simulink model "Single_Phase_VSR_Simulation"  (R2022b)
settings: Solver=FixedStepDiscrete  StartTime=0.0  StopTime=0.6  FixedStep=1e-6  RelTol=1e-3
libraries: spsSeriesRLCBranchLib x10, spsCurrentMeasurementLib x4, spsMosfetLib x4, slpidlib x3, spsRMSLib x3, simulink x3, spsVoltageMeasurementLib x3, spsFourierLib x2, spsMeanLib x2, spsIdealSwitchLib x1, spspowerguiLib x1, spsControlledVoltageSourceLib x1
(part 1 of 2)
settings Model: Creator=XIAO  LastModifiedBy=XIAO
settings SolverCC: AutoInsertRateTranBlk=on
settings DataIOCC: ReturnWorkspaceOutputs=off

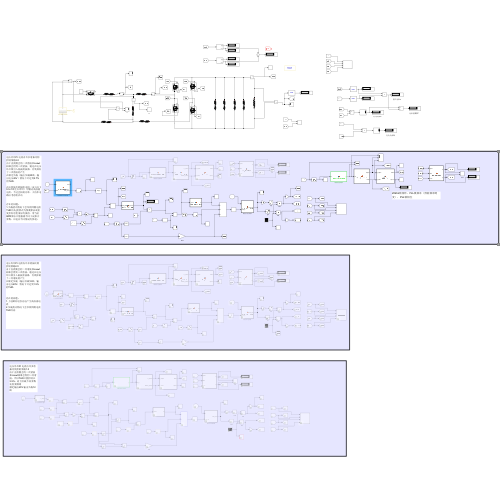
[thumbnail: Simulink's stored preview of the top-level diagram]
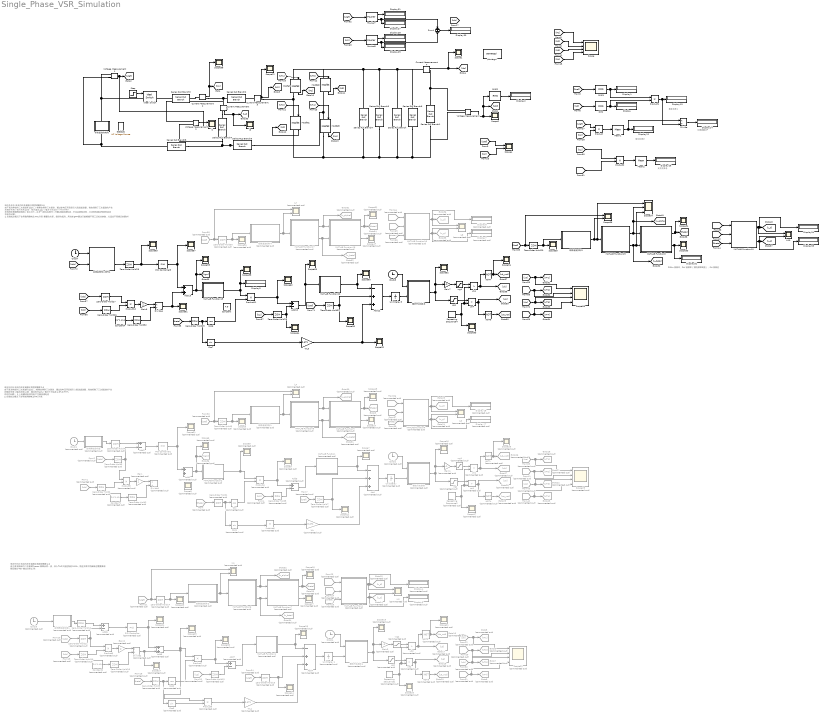
== system Single_Phase_VSR_Simulation ==
  note: 功率因数PF
  note: 有功功率P
  note: 电压外环PI 电流内环多谐振比例控制策略2.0
      | 由于直流侧会的二次谐波和coswt相乘会得到三次谐波，通过在电压环后级引入陷波滤波器，有效抑制了三次谐波的产生
      | 在额定负载（输出负载12欧，输出电压40V）情况下可达到1.5%的THD。
      |
      | 存在的问题：
      | 1.上电瞬间电容充电产生高浪涌电流
      | 2.负载扰动情况下会导致网侧电流THD升高
  note: 无功功率Q
  note: 视在功率s
  note: 电压外环PI 电流内环多谐振比例控制策略1.0
      | 由于直流侧会的二次谐波和coswt相乘会得到三次谐波，所以THD只能控制在3.5%，而且负载不同参数还需要微调
      | 额定输出40V 输出负载12欧
  note: 电压外环PI 电流内环多谐振比例控制策略3.0
      | 由于直流侧会的二次谐波和coswt相乘会得到三次谐波，通过在电压环后级引入陷波滤波器，有效抑制了三次谐波的产生
      | 在额定负载（输出负载20欧，输出电压40V）情况下可达到2.7%的THD。
      |
      | 在电网处串联限流电阻（该工况下0.5~1欧左右即可）可解决高浪涌电流，不过会损耗功率，大功率电路应考虑软启动
      |
      | 存在的问题：
      | 1.负载扰动情况下会导致网侧电流THD升高(需要改为预测算法或重复控制才能很好的抵消，用当前QPR算法只能根据不同工况拟合参数，以适应不同情况的要求)
  note: 20khz锁相环，FLL锁频率（预防频率畸变），PLL锁相位
  -ug1 : Saturate  Commented=on  UpperLimit=1  LowerLimit=-1
  -ug2 : Saturate  Commented=on  UpperLimit=1  LowerLimit=-1
  -ug4 : Saturate  UpperLimit=1  LowerLimit=-1
  Add : Sum  Commented=on  Inputs=-++
  Add1 : Sum  Commented=on
  Add10 : Sum  Inputs=+-
  Add12 : Sum  Inputs=-++
  Add13 : Sum
  Add{2..3,6..7} (4 alike) : Sum  Commented=on  Inputs=+-
  Add4 : Sum  Commented=on  Inputs=-++
  Add5 : Sum  Commented=on
  Clock{1..4} (4 alike) : Clock  Commented=on
  Clock7 : Clock
  Clock8 : Clock
  Constant : Constant  Value=4.9
  Constant1 : Constant  Commented=on  Value=24*1.414
  Constant2 : Constant  Commented=on  Value=24*1.414
  Constant4 : Constant  Value=24*1.414
  Cos : Trigonometry  Commented=on  Operator=cos
  Cos1 : Trigonometry  Commented=on
  Cos2 : Trigonometry  Commented=on  Operator=cos
  Cos3 : Trigonometry  Commented=on
  Cos6 : Trigonometry  Operator=cos
  Cos7 : Trigonometry
  Current Measurement{1..4} (4 alike) : spsCurrentMeasurementLib/Current Measurement  PhasorSimulation=off  OutputType=Complex  PSBequivalent=0
  Display{,1..2,5,12..14,26..34} (16 alike) : Display
  Display{3..4,7..8,17..18} (6 alike) : Display  Commented=on
  Divide : Product  Inputs=*/
  Divide1 : Product  Commented=on  Inputs=*/
  Divide2 : Product  Commented=on  Inputs=*/
  Divide4 : Product  Inputs=*/
  Fourier7 : spsFourierLib/Fourier  Freq=50  n=1  InInit=[0, 0]  Ts=1e-6
  Fourier8 : spsFourierLib/Fourier  Freq=50  n=1  InInit=[0, 0]  Ts=1e-6
  From{,18,25,39,66} (5 alike) : From  Commented=on  GotoTag=theta
  From1 : From  Commented=on  GotoTag=Idc
  From19 : From  Commented=on  GotoTag=Idc
  From2 : From  Commented=on  GotoTag=Udc
  From20 : From  Commented=on  GotoTag=Udc
  From{7,21,30,34,58} (5 alike) : From  Commented=on  GotoTag=Uref
  From22 : From  Commented=on  GotoTag=ua
  From23 : From  Commented=on  GotoTag=u_alpha
  From24 : From  Commented=on  GotoTag=u_beta
  From26 : From  Commented=on  GotoTag=IL2
  From29 : From  Commented=on  GotoTag=ua_not
  From31 : From  Commented=on  GotoTag=ub_not
  From32 : From  Commented=on  GotoTag=ub
  From33 : From  Commented=on  GotoTag=ua
  From36 : From  Commented=on  GotoTag=u_alpha
  From37 : From  Commented=on  GotoTag=u_beta
  From4 : From  Commented=on  GotoTag=IL2
  From41 : From  Commented=on  GotoTag=ua_not
  From42 : From  Commented=on  GotoTag=ub_not
  From43 : From  Commented=on  GotoTag=ub
  From64 : From  Commented=on  GotoTag=u_alpha
  From65 : From  Commented=on  GotoTag=u_beta
  Gain : Gain  Commented=on  Gain=2
  Gain1 : Gain  Commented=on  Gain=-1
  Gain2 : Gain  Commented=on  Gain=2
  Gain3 : Gain  Commented=on  Gain=-1
  Gain6 : Gain  Gain=2
  Gain7 : Gain  Gain=-1
  Goto14 : Goto  Commented=on  GotoTag=u_q
  Goto15 : Goto  Commented=on  GotoTag=u_d
  Goto16 : Goto  Commented=on  GotoTag=ub_not
  Goto17 : Goto  Commented=on  GotoTag=ub
  Goto18 : Goto  Commented=on  GotoTag=VT1
  Goto19 : Goto  Commented=on  GotoTag=ua
  Goto20 : Goto  Commented=on  GotoTag=ua_not
  Goto21 : Goto  Commented=on  GotoTag=VT2
  Goto22 : Goto  Commented=on  GotoTag=VT3
  Goto23 : Goto  Commented=on  GotoTag=VT4
  Goto24 : Goto  Commented=on  GotoTag=u_q
  Goto25 : Goto  Commented=on  GotoTag=u_d
  Goto26 : Goto  Commented=on  GotoTag=ub_not
  Goto27 : Goto  Commented=on  GotoTag=ub
  Goto28 : Goto  Commented=on  GotoTag=ua
  Goto29 : Goto  Commented=on  GotoTag=ua_not
  Goto30 : Goto  Commented=on  GotoTag=u_alpha
  Goto31 : Goto  Commented=on  GotoTag=u_beta
  Goto32 : Goto  Commented=on  GotoTag=u_alpha
  Goto34 : Goto  Commented=on  GotoTag=u_beta
  Goto35 : Goto  Commented=on  GotoTag=theta
  Goto36 : Goto  Commented=on  GotoTag=Igm
  Goto5 : Goto  Commented=on  GotoTag=VT1
  Goto55 : Goto  Commented=on  GotoTag=u_q
  Goto56 : Goto  Commented=on  GotoTag=u_d
  Goto6 : Goto  Commented=on  GotoTag=VT2
  Goto61 : Goto  Commented=on  GotoTag=u_alpha
  Goto62 : Goto  Commented=on  GotoTag=u_beta
  Goto64 : Goto  Commented=on  GotoTag=theta
  Goto7 : Goto  Commented=on  GotoTag=VT3
  Goto8 : Goto  Commented=on  GotoTag=VT4
  Goto9 : Goto  Commented=on  GotoTag=theta
  Ideal Switch : spsIdealSwitchLib/Ideal Switch  Ron=0.001  Lon=0  IC=0  Rs=1e5  Cs=inf  Measurements=on
  MATLAB Function : MATLAB Function  Commented=on  TreatAsAtomicUnit=on
  MATLAB Function1 : MATLAB Function  Commented=on  TreatAsAtomicUnit=on
  MATLAB Function10 : MATLAB Function  TreatAsAtomicUnit=on
  MATLAB Function15 : MATLAB Function  TreatAsAtomicUnit=on
  MATLAB Function16 : MATLAB Function  Commented=on  TreatAsAtomicUnit=on
  MATLAB Function17 : MATLAB Function  Commented=on  TreatAsAtomicUnit=on
  MATLAB Function18 : MATLAB Function  Commented=on  TreatAsAtomicUnit=on
  MATLAB Function19 : MATLAB Function  TreatAsAtomicUnit=on
  MATLAB Function2 : MATLAB Function  Commented=on  TreatAsAtomicUnit=on
  MATLAB Function20 : MATLAB Function  TreatAsAtomicUnit=on
  MATLAB Function3 : MATLAB Function  TreatAsAtomicUnit=on
  MATLAB Function4 : MATLAB Function  Commented=on  TreatAsAtomicUnit=on
  MATLAB Function5 : MATLAB Function  Commented=on  TreatAsAtomicUnit=on
  MATLAB Function6 : MATLAB Function  Commented=on  TreatAsAtomicUnit=on
  MATLAB Function7 : MATLAB Function  Commented=on  TreatAsAtomicUnit=on
  MATLAB Function8 : MATLAB Function  Commented=on  TreatAsAtomicUnit=on
  MATLAB Function9 : MATLAB Function  Commented=on  TreatAsAtomicUnit=on
  Mean1 : spsMeanLib/Mean  Freq=50  Vinit=0  Ts=5e-5
  Mean2 : spsMeanLib/Mean  Freq=50  Vinit=0  Ts=5e-5
  Mosfet{,1..3} (4 alike) : spsMosfetLib/Mosfet  Ron=0.1  Lon=0  Rd=0.01  Vfd=0  IC=0  Rs=1e5  Cs=inf  Measurements=on
  NOT{1..4} (4 alike) : Logic  Commented=on  Operator=NOT  IconShape=distinctive  AllPortsSameDT=off  OutDataTypeStr=boolean
  NOT7 : Logic  Operator=NOT  IconShape=distinctive  AllPortsSameDT=off  OutDataTypeStr=boolean
  NOT8 : Logic  Operator=NOT  IconShape=distinctive  AllPortsSameDT=off  OutDataTypeStr=boolean
  PID Controller : slpidlib/PID Controller  Commented=on  Controller=PI  Form=Parallel  TimeDomain=Discrete-time  UseExternalTs=off  SampleTime=-1  IntegratorMethod=Forward Euler  FilterMethod=Forward Euler  ControllerParametersSource=internal  P=0.5  I=10  UseKiTs=off  D=0  N=100  UseFilter=on  TunerSelectOption=Transfer Function Based (PID Tuner App)  InitialConditionSource=internal  InitialConditionForIntegrator=0  InitialConditionForFilter=0  DifferentiatorICPrevScaledInput=0  ExternalReset=none  TrackingMode=off  Kt=1  LimitOutput=off  SatLimitsSource=internal  UpperSaturationLimit=inf  LowerSaturationLimit=-inf  LinearizeAsGain=on  AntiWindupMode=none  Kb=1  LimitIntegrator=off  UpperIntegratorSaturationLimit=inf  LowerIntegratorSaturationLimit=-inf  POutMin=[]  POutMax=[]  IOutMin=[]  IOutMax=[]  DOutMin=[]  DOutMax=[]  NOutMin=[]  NOutMax=[]  SumOutMin=[]  SumOutMax=[]  SaturationOutMin=[]  SaturationOutMax=[]  PParamMin=[]  PParamMax=[]  IParamMin=[]  IParamMax=[]  DParamMin=[]  DParamMax=[]  NParamMin=[]  NParamMax=[]  KbParamMin=[]  KbParamMax=[]  KtParamMin=[]  KtParamMax=[]  KbOutMin=[]  KbOutMax=[]  KtOutMin=[]  KtOutMax=[]  IntegratorOutMin=[]  IntegratorOutMax=[]  FilterOutMin=[]  FilterOutMax=[]  SumI1OutMin=[]  SumI1OutMax=[]  SumI2OutMin=[]  SumI2OutMax=[]  SumI3OutMin=[]  SumI3OutMax=[]  SumI4OutMin=[]  SumI4OutMax=[]  SumDOutMin=[]  SumDOutMax=[]  DifferentiatorOutMin=[]  DifferentiatorOutMax=[]  FilterDiffOutCoefMin=[]  FilterDiffOutCoefMax=[]  ReciprocalOutMin=[]  ReciprocalOutMax=[]  SumDenOutMin=[]  SumDenOutMax=[]  SumNumOutMin=[]  SumNumOutMax=[]  DivideOutMin=[]  DivideOutMax=[]  UdiffTsProdOutMin=[]  UdiffTsProdOutMax=[]  NTsProdOutMin=[]  NTsProdOutMax=[]  UintegralTsProdOutMin=[]  UintegralTsProdOutMax=[]  UngainTsProdOutMin=[]  UngainTsProdOutMax=[]  ClampingZeroOutDataTypeStr=Inherit: Inherit via back propagation  ClampingZeroOutMin=[]  ClampingZeroOutMax=[]  FilterDenConstantOutDataTypeStr=Inherit: Inherit via back propagation  FilterDenConstantOutMin=[]  FilterDenConstantOutMax=[]  PCopyOutDataTypeStr=Inherit: Inherit via back propagation  PCopyOutMin=[]  PCopyOutMax=[]  NCopyOutDataTypeStr=Inherit: Inherit via back propagation  NCopyOutMin=[]  NCopyOutMax=[]  IntegratorContinuousStateAttributes=''  IntegratorStateMustResolveToSignalObject=off  IntegratorRTWStateStorageClass=Auto  FilterContinuousStateAttributes=''  FilterStateMustResolveToSignalObject=off  FilterRTWStateStorageClass=Auto  ParallelPVariant=InternalParameters  IdealPVariant=Disabled  IVariant=InternalParameters  DVariant=Disabled  IntegratorVariant=Discrete  SatVariant=Disabled  AWVariant=Passthrough  PCopyVariant=Disabled  TRVariant=Disabled  FdbkBlocksVariant=Forward  IdealPFdbkVariant=Disabled  SatFdbkVariant=Disabled  DerivativeFilterVariant=Disabled  NVariant=Disabled  NCopyVariant=Disabled_SignalSpec  FilterICVariant=Disabled  IntegratorICVariant=InternalICs  ExternalResetVariant=Disabled  TRSumVariant=Passthrough  SumFdbkVariant=Disabled  SumVariant=Sum_PI  TsampFilterVariant=InternalTs  TsampNgainVariant=Passthrough  TsampIntegralVariant=Passthrough  ExternalSaturationOutDataTypeStr=Inherit: Same as second input
  PID Controller1 : slpidlib/PID Controller  Commented=on  Controller=PI  Form=Parallel  TimeDomain=Discrete-time  UseExternalTs=off  SampleTime=-1  IntegratorMethod=Forward Euler  FilterMethod=Forward Euler  ControllerParametersSource=internal  P=0.5  I=10  UseKiTs=off  D=0  N=100  UseFilter=on  TunerSelectOption=Transfer Function Based (PID Tuner App)  InitialConditionSource=internal  InitialConditionForIntegrator=0  InitialConditionForFilter=0  DifferentiatorICPrevScaledInput=0  ExternalReset=none  TrackingMode=off  Kt=1  LimitOutput=off  SatLimitsSource=internal  UpperSaturationLimit=inf  LowerSaturationLimit=-inf  LinearizeAsGain=on  AntiWindupMode=none  Kb=1  LimitIntegrator=off  UpperIntegratorSaturationLimit=inf  LowerIntegratorSaturationLimit=-inf  POutMin=[]  POutMax=[]  IOutMin=[]  IOutMax=[]  DOutMin=[]  DOutMax=[]  NOutMin=[]  NOutMax=[]  SumOutMin=[]  SumOutMax=[]  SaturationOutMin=[]  SaturationOutMax=[]  PParamMin=[]  PParamMax=[]  IParamMin=[]  IParamMax=[]  DParamMin=[]  DParamMax=[]  NParamMin=[]  NParamMax=[]  KbParamMin=[]  KbParamMax=[]  KtParamMin=[]  KtParamMax=[]  KbOutMin=[]  KbOutMax=[]  KtOutMin=[]  KtOutMax=[]  IntegratorOutMin=[]  IntegratorOutMax=[]  FilterOutMin=[]  FilterOutMax=[]  SumI1OutMin=[]  SumI1OutMax=[]  SumI2OutMin=[]  SumI2OutMax=[]  SumI3OutMin=[]  SumI3OutMax=[]  SumI4OutMin=[]  SumI4OutMax=[]  SumDOutMin=[]  SumDOutMax=[]  DifferentiatorOutMin=[]  DifferentiatorOutMax=[]  FilterDiffOutCoefMin=[]  FilterDiffOutCoefMax=[]  ReciprocalOutMin=[]  ReciprocalOutMax=[]  SumDenOutMin=[]  SumDenOutMax=[]  SumNumOutMin=[]  SumNumOutMax=[]  DivideOutMin=[]  DivideOutMax=[]  UdiffTsProdOutMin=[]  UdiffTsProdOutMax=[]  NTsProdOutMin=[]  NTsProdOutMax=[]  UintegralTsProdOutMin=[]  UintegralTsProdOutMax=[]  UngainTsProdOutMin=[]  UngainTsProdOutMax=[]  ClampingZeroOutDataTypeStr=Inherit: Inherit via back propagation  ClampingZeroOutMin=[]  ClampingZeroOutMax=[]  FilterDenConstantOutDataTypeStr=Inherit: Inherit via back propagation  FilterDenConstantOutMin=[]  FilterDenConstantOutMax=[]  PCopyOutDataTypeStr=Inherit: Inherit via back propagation  PCopyOutMin=[]  PCopyOutMax=[]  NCopyOutDataTypeStr=Inherit: Inherit via back propagation  NCopyOutMin=[]  NCopyOutMax=[]  IntegratorContinuousStateAttributes=''  IntegratorStateMustResolveToSignalObject=off  IntegratorRTWStateStorageClass=Auto  FilterContinuousStateAttributes=''  FilterStateMustResolveToSignalObject=off  FilterRTWStateStorageClass=Auto  ParallelPVariant=InternalParameters  IdealPVariant=Disabled  IVariant=InternalParameters  DVariant=Disabled  IntegratorVariant=Discrete  SatVariant=Disabled  AWVariant=Passthrough  PCopyVariant=Disabled  TRVariant=Disabled  FdbkBlocksVariant=Forward  IdealPFdbkVariant=Disabled  SatFdbkVariant=Disabled  DerivativeFilterVariant=Disabled  NVariant=Disabled  NCopyVariant=Disabled_SignalSpec  FilterICVariant=Disabled  IntegratorICVariant=InternalICs  ExternalResetVariant=Disabled  TRSumVariant=Passthrough  SumFdbkVariant=Disabled  SumVariant=Sum_PI  TsampFilterVariant=InternalTs  TsampNgainVariant=Passthrough  TsampIntegralVariant=Passthrough  ExternalSaturationOutDataTypeStr=Inherit: Same as second input
  PID Controller3 : slpidlib/PID Controller  Controller=PI  Form=Parallel  TimeDomain=Discrete-time  UseExternalTs=off  SampleTime=-1  IntegratorMethod=Forward Euler  FilterMethod=Forward Euler  ControllerParametersSource=internal  P=0.5  I=10  UseKiTs=off  D=0  N=100  UseFilter=on  TunerSelectOption=Transfer Function Based (PID Tuner App)  InitialConditionSource=internal  InitialConditionForIntegrator=0  InitialConditionForFilter=0  DifferentiatorICPrevScaledInput=0  ExternalReset=none  TrackingMode=off  Kt=1  LimitOutput=off  SatLimitsSource=internal  UpperSaturationLimit=inf  LowerSaturationLimit=-inf  LinearizeAsGain=on  AntiWindupMode=none  Kb=1  LimitIntegrator=off  UpperIntegratorSaturationLimit=inf  LowerIntegratorSaturationLimit=-inf  POutMin=[]  POutMax=[]  IOutMin=[]  IOutMax=[]  DOutMin=[]  DOutMax=[]  NOutMin=[]  NOutMax=[]  SumOutMin=[]  SumOutMax=[]  SaturationOutMin=[]  SaturationOutMax=[]  PParamMin=[]  PParamMax=[]  IParamMin=[]  IParamMax=[]  DParamMin=[]  DParamMax=[]  NParamMin=[]  NParamMax=[]  KbParamMin=[]  KbParamMax=[]  KtParamMin=[]  KtParamMax=[]  KbOutMin=[]  KbOutMax=[]  KtOutMin=[]  KtOutMax=[]  IntegratorOutMin=[]  IntegratorOutMax=[]  FilterOutMin=[]  FilterOutMax=[]  SumI1OutMin=[]  SumI1OutMax=[]  SumI2OutMin=[]  SumI2OutMax=[]  SumI3OutMin=[]  SumI3OutMax=[]  SumI4OutMin=[]  SumI4OutMax=[]  SumDOutMin=[]  SumDOutMax=[]  DifferentiatorOutMin=[]  DifferentiatorOutMax=[]  FilterDiffOutCoefMin=[]  FilterDiffOutCoefMax=[]  ReciprocalOutMin=[]  ReciprocalOutMax=[]  SumDenOutMin=[]  SumDenOutMax=[]  SumNumOutMin=[]  SumNumOutMax=[]  DivideOutMin=[]  DivideOutMax=[]  UdiffTsProdOutMin=[]  UdiffTsProdOutMax=[]  NTsProdOutMin=[]  NTsProdOutMax=[]  UintegralTsProdOutMin=[]  UintegralTsProdOutMax=[]  UngainTsProdOutMin=[]  UngainTsProdOutMax=[]  ClampingZeroOutDataTypeStr=Inherit: Inherit via back propagation  ClampingZeroOutMin=[]  ClampingZeroOutMax=[]  FilterDenConstantOutDataTypeStr=Inherit: Inherit via back propagation  FilterDenConstantOutMin=[]  FilterDenConstantOutMax=[]  PCopyOutDataTypeStr=Inherit: Inherit via back propagation  PCopyOutMin=[]  PCopyOutMax=[]  NCopyOutDataTypeStr=Inherit: Inherit via back propagation  NCopyOutMin=[]  NCopyOutMax=[]  IntegratorContinuousStateAttributes=''  IntegratorStateMustResolveToSignalObject=off  IntegratorRTWStateStorageClass=Auto  FilterContinuousStateAttributes=''  FilterStateMustResolveToSignalObject=off  FilterRTWStateStorageClass=Auto  ParallelPVariant=InternalParameters  IdealPVariant=Disabled  IVariant=InternalParameters  DVariant=Disabled  IntegratorVariant=Discrete  SatVariant=Disabled  AWVariant=Passthrough  PCopyVariant=Disabled  TRVariant=Disabled  FdbkBlocksVariant=Forward  IdealPFdbkVariant=Disabled  SatFdbkVariant=Disabled  DerivativeFilterVariant=Disabled  NVariant=Disabled  NCopyVariant=Disabled_SignalSpec  FilterICVariant=Disabled  IntegratorICVariant=InternalICs  ExternalResetVariant=Disabled  TRSumVariant=Passthrough  SumFdbkVariant=Disabled  SumVariant=Sum_PI  TsampFilterVariant=InternalTs  TsampNgainVariant=Passthrough  TsampIntegralVariant=Passthrough  ExternalSaturationOutDataTypeStr=Inherit: Same as second input
  Product{,1..2,11..12} (5 alike) : Product
  Product{3..8} (6 alike) : Product  Commented=on
  RMS : spsRMSLib/RMS  TrueRMS=on  Freq=50  RMSInit=24  Ts=1e-6
  RMS1 : spsRMSLib/RMS  TrueRMS=on  Freq=50  RMSInit=24  Ts=1e-6
  RMS2 : spsRMSLib/RMS  TrueRMS=on  Freq=50  RMSInit=24  Ts=1e-6
  Repeating Sequence1 : simulink/Sources/Repeating Sequence  Commented=on  rep_seq_t=[0, 5e-5, 1e-4]  rep_seq_y=[-1, 1, -1]
  Repeating Sequence2 : simulink/Sources/Repeating Sequence  Commented=on  rep_seq_t=[0, 5e-5, 1e-4]  rep_seq_y=[-1, 1, -1]
  Repeating Sequence4 : simulink/Sources/Repeating Sequence  rep_seq_t=[0, 5e-5, 1e-4]  rep_seq_y=[-1, 1, -1]
  Scope : Scope  NumInputPorts=4
  Scope{1..2,12,32..35,38,50,52,54,57..65} (20 alike) : Scope
  Scope{3,5..11,13..16,18..19,21,23..28,30..31,49,51,56} (26 alike) : Scope  Commented=on
  Scope17 : Scope  Commented=on  NumInputPorts=2
  Scope20 : Scope  Commented=on  NumInputPorts=2
  Scope22 : Scope  Commented=on  NumInputPorts=4
  Scope29 : Scope  Commented=on  NumInputPorts=4
  Scope36 : Scope  NumInputPorts=2
  Scope37 : Scope  NumInputPorts=3
  Scope4 : Scope  NumInputPorts=2
  Scope53 : Scope  NumInputPorts=2
  Scope55 : Scope  NumInputPorts=4
  Series RLC Branch{,5..7} (4 alike) : spsSeriesRLCBranchLib/Series RLC Branch  LConnTagsString=__new0  RConnTagsString=__new0  BranchType=RC  Resistance=0.01  Inductance=0  SetiL0=off  InitialCurrent=0  Capacitance=470e-6  Setx0=off  InitialVoltage=0  Measurements=None
  Series RLC Branch1 : spsSeriesRLCBranchLib/Series RLC Branch  LConnTagsString=__new0  RConnTagsString=__new0  BranchType=R  Resistance=20  Inductance=0  SetiL0=off  InitialCurrent=0  Capacitance=470e-6  Setx0=off  InitialVoltage=0  Measurements=None
  Series RLC Branch2 : spsSeriesRLCBranchLib/Series RLC Branch  LConnTagsString=__new0  RConnTagsString=__new0  BranchType=RL  Resistance=0.1  Inductance=0.0015  SetiL0=off  InitialCurrent=0  Capacitance=220e-6  Setx0=off  InitialVoltage=0  Measurements=None
  Series RLC Branch3 : spsSeriesRLCBranchLib/Series RLC Branch  LConnTagsString=__new0  RConnTagsString=__new0  BranchType=RL  Resistance=0.1  Inductance=0.00012  SetiL0=off  InitialCurrent=0  Capacitance=220e-6  Setx0=off  InitialVoltage=0  Measurements=None
  Series RLC Branch4 : spsSeriesRLCBranchLib/Series RLC Branch  LConnTagsString=__new0  RConnTagsString=__new0  BranchType=RC  Resistance=0.1  Inductance=0  SetiL0=off  InitialCurrent=0  Capacitance=10e-6  Setx0=off  InitialVoltage=0  Measurements=None
  Series RLC Branch8 : spsSeriesRLCBranchLib/Series RLC Branch  LConnTagsString=__new0  RConnTagsString=__new0  BranchType=RL  Resistance=0.1  Inductance=0.00012  SetiL0=off  InitialCurrent=0  Capacitance=220e-6  Setx0=off  InitialVoltage=0  Measurements=None
  Series RLC Branch9 : spsSeriesRLCBranchLib/Series RLC Branch  LConnTagsString=__new0  RConnTagsString=__new0  BranchType=RL  Resistance=0.1  Inductance=0.0015  SetiL0=off  InitialCurrent=0  Capacitance=220e-6  Setx0=off  InitialVoltage=0  Measurements=None
  Step : Step  Time=0.15  SampleTime=1e-6
  Sum4 : Sum  Inputs=+-
  Unit Delay : UnitDelay  Commented=on  SampleTime=5e-5  HasFrameUpgradeWarning=on
  Unit Delay1 : UnitDelay  Commented=on  SampleTime=5e-5  HasFrameUpgradeWarning=on
  Unit Delay3 : UnitDelay  SampleTime=5e-5  HasFrameUpgradeWarning=on
  Voltage Measurement : spsVoltageMeasurementLib/Voltage Measurement  PhasorSimulation=off  OutputType=Complex  PSBequivalent=0
  Voltage Measurement1 : spsVoltageMeasurementLib/Voltage Measurement  PhasorSimulation=off  OutputType=Complex  PSBequivalent=0
  Voltage Measurement2 : spsVoltageMeasurementLib/Voltage Measurement  PhasorSimulation=off  OutputType=Complex  PSBequivalent=0
  WL : Gain  Commented=on  Gain=0.471
  WL1 : Gain  Commented=on  Gain=0.471
  WL3 : Gain  Gain=0.471
  Zero-Order Hold{1..5,7..13,15..16} (14 alike) : ZeroOrderHold  Commented=on  SampleTime=5e-5
  Zero-Order Hold14 : ZeroOrderHold  Commented=on  SampleTime=1e-5
  Zero-Order Hold{20,25..29,31..32} (8 alike) : ZeroOrderHold  SampleTime=5e-5
  Zero-Order Hold30 : ZeroOrderHold  Commented=on  SampleTime=1e-5
  Zero-Order Hold6 : ZeroOrderHold  Commented=on  SampleTime=1e-5
  i1 : Scope  NumInputPorts=2
  i3 : Scope
  iL{1..2,4..5,7..8} (6 alike) : Scope  Commented=on  NumInputPorts=2
  iL10 : Scope  NumInputPorts=2
  powergui : spspowerguiLib/powergui  Priority=1  SimulationMode=Discrete  SampleTime=1e-6  frequency=60  Iterations=50  frequencyindice=0  Pbase=100e6  ErrMax=1e-4  UnitsV=kV  UnitsW=MW  buscounter=0  FunctionMessages=off  echomessages=off  EnableUseOfTLC=off  CurrentSourceSwitches=off  DisableSnubberDevices=off  DisableRonSwitches=off  DisableVfSwitches=off  DisplayEquations=off  AutomaticDiscreteSolvers=off  SolverType=Tustin/Backward Euler (TBE)  Interpol=off  ExternalGateDelay=off  methode=off  Ts=100  x0status=blocks  SPID=on  SwTol=0  HookPort=off  NonlinearTolerance=1e-4  nMaxIteration=100  ContinueOnMaxIteration=off  RestoreLinks=warning  ResistiveCurrentMeasurement=off  Frange=[0:2:500]  Ylog=off  Xlog=on  ShowGrid=off  save=off  variable=ZData  structure=0  ZoomFFT=off  StartTime=0.0  cycles=1  DisplayStyle=1  fundamental=60  FreqAxis=off  MaxFrequency=1000  frequencyindicesteady=1  RmsSteady=1  display=off
  ua1 : RelationalOperator  Commented=on  Operator=>  OutDataTypeStr=boolean  RndMeth=Simplest  InputSameDT=off
  ua2 : RelationalOperator  Commented=on  Operator=>  OutDataTypeStr=boolean  RndMeth=Simplest  InputSameDT=off
  ua4 : RelationalOperator  Operator=>  OutDataTypeStr=boolean  RndMeth=Simplest  InputSameDT=off
  ub1 : RelationalOperator  Commented=on  Operator=>  OutDataTypeStr=boolean  RndMeth=Simplest  InputSameDT=off
  ub2 : RelationalOperator  Commented=on  Operator=>  OutDataTypeStr=boolean  RndMeth=Simplest  InputSameDT=off
  ub4 : RelationalOperator  Operator=>  OutDataTypeStr=boolean  RndMeth=Simplest  InputSameDT=off
  ug1 : Saturate  Commented=on  UpperLimit=1  LowerLimit=-1
  ug2 : Saturate  Commented=on  UpperLimit=1  LowerLimit=-1
  ug4 : Saturate  UpperLimit=1  LowerLimit=-1
  合闸再给目标值 : MATLAB Function  Commented=on  TreatAsAtomicUnit=on
  合闸再给目标值1 : MATLAB Function  Commented=on  TreatAsAtomicUnit=on
  合闸后再传入信号1 : MATLAB Function  TreatAsAtomicUnit=on
  带有谐波的电网 : Subsystem
  模仿开关控制 : MATLAB Function  Commented=on  TreatAsAtomicUnit=on
  模仿开关控制1 : MATLAB Function  Commented=on  TreatAsAtomicUnit=on
  模仿开关控制3 : MATLAB Function  TreatAsAtomicUnit=on
  理想电网 : spsACVoltageSourceLib/AC Voltage Source  Amplitude=24*1.414  Phase=0  Frequency=50  SampleTime=0  Measurements=None  BusType=swing  Pref=10e3  Qref=0  Qmin=-inf  Qmax=+inf
  级联谐波抑制1 : MATLAB Function  Commented=on  TreatAsAtomicUnit=on
  级联谐波抑制2 : MATLAB Function  Commented=on  TreatAsAtomicUnit=on
  级联谐波抑制3 : MATLAB Function  TreatAsAtomicUnit=on
  级联谐波抑制4 : MATLAB Function  Commented=on  TreatAsAtomicUnit=on
  wires:
  Repeating Sequence2/1 -> ub1/2, ua1/2, Scope17/1
  [Uref] -> Fourier7/1
  Mean2/1 -> Display26/1
  Sum4/1 -> Display30/1
  [VT1] -> Mosfet/1
  [IL2] -> Fourier8/1
  Fourier8/2 -> Sum4/2, Display29/1
  Fourier8/1 -> Display28/1
  ua1/1 -> Goto28/1, NOT4/1
  [u_beta] -> Product2/2
  Fourier7/2 -> Display27/1, Sum4/1
  [IL2] -> RMS/1
  [IL2] -> Product2/1
  From33/1 -> Scope29/1, Goto18/1
  [M1] -> Scope/1
  Product2/1 -> Mean2/1
  From36/1 -> MATLAB Function5/1(alpha)
  [Uref] -> Product/1
  Mosfet3/1 -> [M4]
  From43/1 -> Scope29/3, Goto22/1
  [M4] -> Scope/4
  RMS1/1 -> Product1/1, Display1/1
  Gain1/1 -> -ug1/1
  Product1/1 -> Divide/2, Display13/1
  MATLAB Function9/2(qerror) -> Scope10/1
  Divide/1 -> Display14/1
  Mosfet2/1 -> [M3]
  [VT4] -> Mosfet3/1
  ug1/1 -> ua1/1
  Mean1/1 -> Divide/1, Display12/1
  Mosfet/1 -> [M1]
  Mosfet1/1 -> [M2]
  [M3] -> Scope/3
  [VT2] -> Mosfet1/1
  RMS/1 -> Product1/2, Display/1
  [Uref] -> RMS1/1
  NOT1/1 -> Scope28/1, Goto26/1
  [VT3] -> Mosfet2/1
  Fourier7/1 -> Display31/1
  Voltage Measurement1/1 -> i1/2, [Uref]
  级联谐波抑制1/1(y) -> iL4/2, MATLAB Function8/1(U_in)
  -ug1/1 -> ub1/1
  From41/1 -> Scope29/2, Goto21/1
  From42/1 -> Scope29/4, Goto23/1
  ub1/1 -> Goto27/1, NOT1/1
  MATLAB Function5/2(q) -> Display17/1, Goto24/1, iL5/2
  MATLAB Function8/2(deltaU_prime) -> Goto31/1, MATLAB Function9/2(u_beta)
  Product/1 -> Mean1/1
  NOT4/1 -> Goto29/1
  [M2] -> Scope/2
  Current Measurement1/1 -> i3/1, [I_c]
  [IL2] -> Product/2
  From30/1 -> iL4/1, Zero-Order Hold6/1
  MATLAB Function8/1(U_prime) -> MATLAB Function9/1(u_alpha), Goto30/1
  From37/1 -> MATLAB Function5/2(beta)
  From39/1 -> MATLAB Function5/3(theta)
  MATLAB Function5/1(d) -> iL5/1, Display18/1, Goto25/1
  Zero-Order Hold6/1 -> 级联谐波抑制1/1(u), Scope3/1
  MATLAB Function9/1(theta) -> Scope15/1, Goto9/1
  Voltage Measurement/1 -> [Udc], RMS2/1, Scope2/1
  RMS2/1 -> Display2/1
  Current Measurement2/1 -> Scope38/1, [IL1]
  Current Measurement3/1 -> [IL2], Scope12/1
  From/1 -> Zero-Order Hold1/1
  Zero-Order Hold1/1 -> Cos1/1, Cos/1
  Current Measurement4/1 -> Scope1/1, [Idc]
  From1/1 -> Zero-Order Hold2/1
  From2/1 -> Zero-Order Hold3/1
  Zero-Order Hold4/1 -> Add2/1
  Zero-Order Hold3/1 -> Product3/1, Add2/2
  Zero-Order Hold2/1 -> Product3/2
  Product3/1 -> Gain/1
  Gain/1 -> Divide1/1
  Cos/1 -> Product4/2
  Product4/1 -> Scope9/1, Add3/1
  From4/1 -> Zero-Order Hold5/1
  Zero-Order Hold5/1 -> Add3/2
  Add3/1 -> MATLAB Function/1(i_error)
  From7/1 -> Zero-Order Hold7/1
  Zero-Order Hold7/1 -> Add/2, Scope11/1
  Cos1/1 -> Product5/2
  Product5/1 -> WL/1
  Constant1/1 -> Zero-Order Hold8/1
  Zero-Order Hold8/1 -> Divide1/2
  [IL2] -> Scope4/2
  [Uref] -> Scope4/1
  MATLAB Function/1(m) -> Add/1, Scope7/1
  Step/1 -> Ideal Switch/1
  Clock1/1 -> 合闸再给目标值/1(t)
  合闸再给目标值/1(V_amp) -> Zero-Order Hold4/1
  Clock2/1 -> 模仿开关控制/1(t)
  模仿开关控制/1(mod_out) -> ug1/1, Scope16/1, Gain1/1
  Add/1 -> Unit Delay/1
  Unit Delay/1 -> 模仿开关控制/2(mod_in)
  WL/1 -> Add/3
  Add4/1 -> Unit Delay1/1
  Clock3/1 -> 合闸再给目标值1/1(t)
  Unit Delay1/1 -> 模仿开关控制1/2(mod_in)
  MATLAB Function1/1(m) -> Add4/1, Scope26/1
  模仿开关控制1/1(mod_out) -> ug2/1, Scope19/1, Gain3/1
  合闸再给目标值1/1(V_amp) -> Zero-Order Hold12/1
  Clock4/1 -> 模仿开关控制1/1(t)
  ua2/1 -> Goto19/1, NOT3/1
  MATLAB Function7/1(theta) -> Scope18/1, Goto35/1
  MATLAB Function4/1(d) -> iL2/1, Display4/1, Goto15/1
  Zero-Order Hold13/1 -> Add7/2
  Constant2/1 -> Zero-Order Hold16/1
  Divide2/1 -> Add5/2, Scope27/1
  From23/1 -> MATLAB Function4/1(alpha)
  NOT3/1 -> Goto20/1
  Zero-Order Hold16/1 -> Divide2/2
  Add7/1 -> MATLAB Function1/1(i_error)
  Zero-Order Hold10/1 -> Product6/2
  Product8/1 -> WL1/1
  MATLAB Function6/1(U_prime) -> MATLAB Function7/1(u_alpha), Goto32/1
  From34/1 -> Zero-Order Hold15/1
  Zero-Order Hold9/1 -> Cos3/1, Cos2/1
  Cos2/1 -> Product7/2
  Zero-Order Hold15/1 -> Add4/2, Scope14/1
  ub2/1 -> Goto17/1, NOT2/1
  Zero-Order Hold11/1 -> Product6/1, Add6/2
  From26/1 -> Zero-Order Hold13/1
  From18/1 -> Zero-Order Hold9/1
  Cos3/1 -> Product8/2
  From19/1 -> Zero-Order Hold10/1
  From24/1 -> MATLAB Function4/2(beta)
  Product7/1 -> Scope30/1, Add7/1
  From25/1 -> MATLAB Function4/3(theta)
  From29/1 -> Scope22/2, Goto6/1
  Gain2/1 -> Divide2/1
  NOT2/1 -> Scope21/1, Goto16/1
  级联谐波抑制2/1(y) -> iL1/2, MATLAB Function6/1(U_in)
  Zero-Order Hold12/1 -> Add6/1
  MATLAB Function4/2(q) -> Display3/1, Goto14/1, iL2/2
  From31/1 -> Scope22/4, Goto8/1
  From22/1 -> Scope22/1, Goto5/1
  From21/1 -> iL1/1, Zero-Order Hold14/1
  WL1/1 -> Add4/3
  Product6/1 -> Gain2/1
  From32/1 -> Scope22/3, Goto7/1
  -ug2/1 -> ub2/1
  From20/1 -> Zero-Order Hold11/1
  Gain3/1 -> -ug2/1
  MATLAB Function7/2(qerror) -> Scope13/1
  ug2/1 -> ua2/1
  MATLAB Function6/2(deltaU_prime) -> Goto34/1, MATLAB Function7/2(u_beta)
  Zero-Order Hold14/1 -> 级联谐波抑制2/1(u), Scope23/1
  Repeating Sequence1/1 -> ub2/2, ua2/2, Scope20/1
  Add6/1 -> PID Controller/1
  PID Controller/1 -> Scope24/1, Add5/1
  Add5/1 -> Scope25/1, Product7/1, Product8/1
  Add2/1 -> PID Controller1/1
  PID Controller1/1 -> Scope31/1, Add1/1
  Add1/1 -> MATLAB Function2/1(IGm_total), Scope6/1, Goto36/1
  MATLAB Function2/1(Igm_clean) -> Product4/1, Scope5/1
  Cos7/1 -> WL3/1
  [ub] -> Scope55/3, [VT3]
  Repeating Sequence4/1 -> ub4/2, ua4/2, Scope53/1
  模仿开关控制3/1(mod_out) -> ug4/1, Scope52/1, Gain7/1
  MATLAB Function20/1(m) -> Add12/1, Scope60/1
  [ua] -> Scope55/1, [VT1]
  MATLAB Function17/2(deltaU_prime) -> Goto62/1, MATLAB Function18/2(u_beta)
  MATLAB Function18/2(qerror) -> Scope49/1
  -ug4/1 -> ub4/1
  ug4/1 -> ua4/1
  Add13/1 -> MATLAB Function15/1(IGm_total), Scope59/1, [Igm]
  [ub_not] -> Scope55/4, [VT4]
  Add12/1 -> Unit Delay3/1
  [Udc] -> Zero-Order Hold27/1
  WL3/1 -> Add12/3, Scope32/1
  Product11/1 -> Add10/1, Scope62/1
  NOT7/1 -> Scope54/1, [ub_not]
  MATLAB Function15/1(Igm_clean) -> Product11/1, Scope58/1, Display5/1
  Gain6/1 -> Divide4/1
  Zero-Order Hold27/1 -> Product12/1
  [Idc] -> Zero-Order Hold26/1
  Zero-Order Hold32/1 -> Divide4/2
  Cos6/1 -> Product11/2
  级联谐波抑制4/1(y) -> iL7/2, MATLAB Function17/1(U_in)
  [theta] -> Zero-Order Hold25/1
  Constant4/1 -> Zero-Order Hold32/1
  [IL2] -> Zero-Order Hold29/1
  MATLAB Function17/1(U_prime) -> MATLAB Function18/1(u_alpha), Goto61/1
  Zero-Order Hold31/1 -> Add12/2, Scope50/1
  From64/1 -> MATLAB Function16/1(alpha)
  Zero-Order Hold26/1 -> Product12/2
  ub4/1 -> [ub], NOT7/1
  MATLAB Function16/1(d) -> iL8/1, Display8/1, Goto56/1
  PID Controller3/1 -> Scope57/1, Add13/1
  NOT8/1 -> [ua_not]
  Unit Delay3/1 -> 模仿开关控制3/2(mod_in)
  MATLAB Function18/1(theta) -> Scope51/1, Goto64/1
  From58/1 -> iL7/1, Zero-Order Hold30/1
  From66/1 -> MATLAB Function16/3(theta)
  Clock7/1 -> 合闸后再传入信号1/1(t)
  From65/1 -> MATLAB Function16/2(beta)
  Product12/1 -> Gain6/1
  MATLAB Function16/2(q) -> Display7/1, Goto55/1, iL8/2
  [Uref] -> Zero-Order Hold31/1
  Zero-Order Hold29/1 -> Scope64/1, Add10/2
  Zero-Order Hold28/1 -> PID Controller3/1, Scope63/1
  ua4/1 -> [ua], NOT8/1
  [ua_not] -> Scope55/2, [VT2]
  Clock8/1 -> 模仿开关控制3/1(t)
  Zero-Order Hold30/1 -> 级联谐波抑制4/1(u), Scope56/1
  Add10/1 -> Scope65/1, MATLAB Function20/1(i_error)
  合闸后再传入信号1/2(Udc_error) -> Zero-Order Hold28/1
  [Udc] -> 合闸后再传入信号1/2(Udc)
  Gain7/1 -> -ug4/1
  Zero-Order Hold25/1 -> Cos7/1, Cos6/1
  Voltage Measurement2/1 -> i1/1
  Divide4/1 -> Scope61/1, Add13/2
  MATLAB Function19/1(alpha) -> Scope37/2, [u_alpha], MATLAB Function3/1(u_alpha)
  MATLAB Function19/2(beta) -> Scope37/3, MATLAB Function3/2(u_beta), [u_beta]
  MATLAB Function10/1(d) -> iL10/1, Display34/1, [u_d]
  MATLAB Function3/1(theta) -> Scope34/1, [theta]
  MATLAB Function10/2(q) -> Display33/1, [u_q], iL10/2
  Zero-Order Hold20/1 -> 级联谐波抑制3/1(u), Scope35/1
  [u_alpha] -> MATLAB Function10/1(alpha)
  [theta] -> MATLAB Function10/3(theta)
  [Uref] -> Scope36/1, Zero-Order Hold20/1
  MATLAB Function3/2(qerror) -> Scope33/1, Display32/1
  [u_beta] -> MATLAB Function10/2(beta)
  级联谐波抑制3/1(y) -> Scope36/2, Scope37/1, MATLAB Function19/1(uin)
  connections:
  Current Measurement2/LConn1 -- Series RLC Branch3/LConn1
  Current Measurement1/RConn1 -- Series RLC Branch4/LConn1
  Mosfet3/RConn1 -- Series RLC Branch1/RConn1 -- Voltage Measurement/LConn2 -- Series RLC Branch6/RConn1 -- Series RLC Branch/RConn1 -- Series RLC Branch5/RConn1 -- Series RLC Branch7/RConn1 -- Mosfet1/RConn1
  Current Measurement4/LConn1 -- Series RLC Branch6/LConn1 -- Mosfet/LConn1 -- Mosfet2/LConn1 -- Series RLC Branch7/LConn1 -- Series RLC Branch5/LConn1 -- Series RLC Branch/LConn1
  Mosfet/RConn1 -- Current Measurement3/RConn1 -- Mosfet1/LConn1
  Series RLC Branch9/RConn1 -- Voltage Measurement2/LConn2 -- Series RLC Branch4/RConn1 -- Series RLC Branch8/LConn1
  Current Measurement2/RConn1 -- Current Measurement1/LConn1 -- Voltage Measurement2/LConn1 -- Series RLC Branch2/RConn1
  Current Measurement3/LConn1 -- Series RLC Branch2/LConn1
  Voltage Measurement/LConn1 -- Current Measurement4/RConn1 -- Series RLC Branch1/LConn1
  带有谐波的电网/RConn1 -- Ideal Switch/LConn1 -- Voltage Measurement1/LConn1
  Series RLC Branch3/RConn1 -- Ideal Switch/RConn1
  带有谐波的电网/LConn1 -- Series RLC Branch8/RConn1 -- Voltage Measurement1/LConn2
  Series RLC Branch9/LConn1 -- Mosfet3/LConn1 -- Mosfet2/RConn1

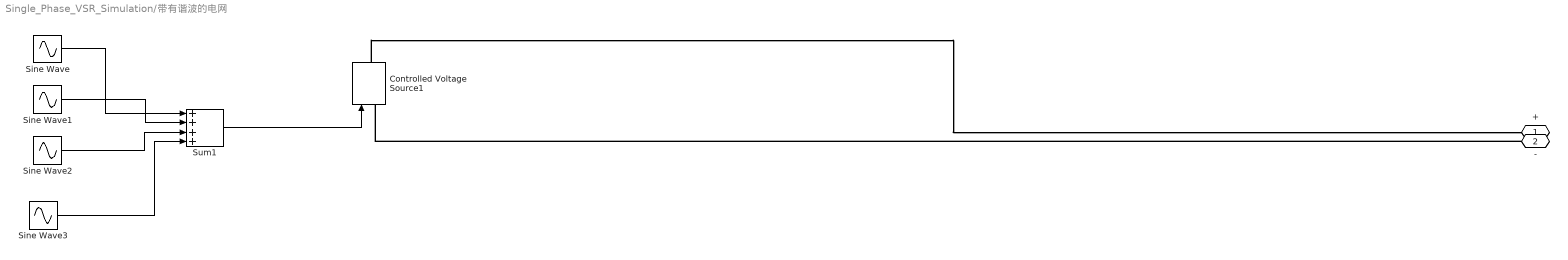
== system Single_Phase_VSR_Simulation/带有谐波的电网 ==
  Controlled Voltage Source1 : spsControlledVoltageSourceLib/Controlled Voltage Source  Initialize=off  Source_Type=AC  Amplitude=0  Phase=0  Frequency=0  Measurements=Voltage
  Sine Wave : Sin  Amplitude=24*sqrt(2)  Frequency=100*pi  SampleTime=0
  Sine Wave1 : Sin  Amplitude=0.04*24*sqrt(2)  Frequency=300*pi  SampleTime=0
  Sine Wave2 : Sin  Amplitude=0.03*24*sqrt(2)  Frequency=500*pi  SampleTime=0
  Sine Wave3 : Sin  Amplitude=0.02*24*sqrt(2)  Frequency=700*pi  SampleTime=0
  Sum1 : Sum  Inputs=++++
  + : PMIOPort  Side=Right
  - : PMIOPort  Port=2  Side=Left
  wires:
  Sum1/1 -> Controlled Voltage Source1/1
  Sine Wave1/1 -> Sum1/2
  Sine Wave/1 -> Sum1/1
  Sine Wave3/1 -> Sum1/4
  Sine Wave2/1 -> Sum1/3
  connections:
  -/RConn1 -- Controlled Voltage Source1/LConn1
  Controlled Voltage Source1/RConn1 -- +/RConn1

== matlab function Single_Phase_VSR_Simulation/MATLAB Function9 ==
  data: u_alpha input; theta output; u_beta input; qerror output
function [theta, qerror] = SRF_PLL(u_alpha, u_beta)
% 同步旋转坐标系锁相环 SRF-PLL（严格匹配框图逻辑）
% 输入
%   u_alpha:  α轴输入信号（对应框图的v'，与电网电压同相）
%   u_beta:   β轴输入信号（对应框图的qv'，与电网电压正交90°）
% 输出
%   theta:    锁相得到的电网相位 [0, 2π)
%   qerror:   q轴相位误差（锁相锁定时趋近于0）
% 适配：仿真步长 Ts=1e-5（10kHz采样），基波频率50Hz

    %% ===================== 1. 固定参数配置 =====================
    Ts = 1e-5;               % 采样时间，必须与全局仿真步长完全一致
    f0 = 50;                  % 电网额定基波频率 (Hz)
    w0 = 2 * pi * f0;        % 额定角频率 (rad/s)
    
    % PI控制器参数（适配10kHz采样，可按需调整）
    kp_pll = 60;              % 比例系数：增大加快锁相响应，过大易振荡
    ki_pll = 5000;            % 积分系数：增大减小稳态相位误差，过大影响稳定性

    %% ===================== 2. 持久变量初始化（仅首次运行执行） =====================
    persistent theta_prev     % 上一拍的锁相相位
    persistent xi_pll         % PI控制器的积分项（抗饱和）
    
    if isempty(theta_prev)
        theta_prev = 0;       % 相位初始值清零
        xi_pll = 0;           % 积分项初始值清零
    end

    %% ===================== 3. αβ/dq 帕克变换（核心鉴相环节） =====================
    % 标准帕克变换矩阵，严格匹配框图逻辑
    % [u_d]   = [ cosθ   sinθ ] [u_alpha]
    % [u_q]     [ -sinθ  cosθ ] [u_beta ]
    cos_theta = cos(theta_prev);
    sin_theta = sin(theta_prev);
    
    u_d = u_alpha * cos_theta + u_beta * sin_theta;  % d轴分量（对应电压幅值）
    u_q = -u_alpha * sin_theta + u_beta * cos_theta; % q轴分量（相位误差）
    
    qerror = u_q; % 输出q轴相位误差，锁相锁定时qerror→0

    %% ===================== 4. PI环路控制器 =====================
    % 位置式PI控制器，带积分抗饱和
    xi_pll = xi_pll + ki_pll * Ts * qerror;  % 积分项更新
    delta_w = kp_pll * qerror + xi_pll;      % 频率偏差量
    w_pll = w0 + delta_w;                     % 锁相得到的实时角频率

    %% ===================== 5. 积分环节（1/s）生成相位 =====================
    % 前向欧拉离散化，对应框图的1/s积分环节
    theta = theta_prev + Ts * w_pll;
    
    % 相位归一化到 [0, 2π)，防止数值溢出
    theta = mod(theta, 2 * pi);

    %% ===================== 6. 更新状态变量（为下一拍迭代准备） =====================
    theta_prev = theta;

end

== matlab function Single_Phase_VSR_Simulation/级联谐波抑制1 ==
  data: u input; y output
function y = Cascade_Notch_Filter(u)
% 级联陷波滤波器：滤除3/5/7次固定频率谐波（150/250/350Hz）
% 输入u：待滤波的标量信号
% 输出y：滤波后的标量信号
% 适配：20kHz采样率（Ts=5e-5），和你的控制环完全对齐

    persistent x3_1 x3_2 x5_1 x5_2 x7_1 x7_2 first_run
    persistent b3_0 b3_1 b3_2 a3_1 a3_2
    persistent b5_0 b5_1 b5_2 a5_1 a5_2
    persistent b7_0 b7_1 b7_2 a7_1 a7_2

    %% ===================== 1. 初始化：仅首次运行 =====================
    if isempty(first_run)
        % --- 固定参数 ---
        Fs = 1e5;          % 采样频率 100kHz
        Ts = 1/Fs;            % 采样周期 5e-5s
        wc = 10;              % 截止角频率 25 rad/s
        
        % 目标谐波频率
        w3 = 2*pi*150;  % 3次谐波 150Hz
        w5 = 2*pi*250;  % 5次谐波 250Hz
        w7 = 2*pi*350;  % 7次谐波 350Hz

        % --- Tustin变换预计算系数 ---
        k = 2/Ts;
        k2 = k*k;

        % --- 3次滤波器系数 ---
        [b3_0, b3_1, b3_2, a3_1, a3_2] = calc_coeff(w3, wc, k, k2);
        % --- 5次滤波器系数 ---
        [b5_0, b5_1, b5_2, a5_1, a5_2] = calc_coeff(w5, wc, k, k2);
        % --- 7次滤波器系数 ---
        [b7_0, b7_1, b7_2, a7_1, a7_2] = calc_coeff(w7, wc, k, k2);

        % --- 显式初始化状态变量为标量 ---
        x3_1 = 0; x3_2 = 0;
        x5_1 = 0; x5_2 = 0;
        x7_1 = 0; x7_2 = 0;
        
        first_run = 1;
    end

    %% ===================== 2. 级联滤波计算（显式差分方程） =====================
    % --- 第1级：3次谐波滤波 ---
    y3 = b3_0*u + x3_1;
    x3_1_next = b3_1*u - a3_1*y3 + x3_2;
    x3_2_next = b3_2*u - a3_2*y3;
    
    % --- 第2级：5次谐波滤波 ---
    y5 = b5_0*y3 + x5_1;
    x5_1_next = b5_1*y3 - a5_1*y5 + x5_2;
    x5_2_next = b5_2*y3 - a5_2*y5;
    
    % --- 第3级：7次谐波滤波 ---
    y7 = b7_0*y5 + x7_1;
    x7_1_next = b7_1*y5 - a7_1*y7 + x7_2;
    x7_2_next = b7_2*y5 - a7_2*y7;
    
    % --- 更新状态变量 ---
    x3_1 = x3_1_next; x3_2 = x3_2_next;
    x5_1 = x5_1_next; x5_2 = x5_2_next;
    x7_1 = x7_1_next; x7_2 = x7_2_next;
    
    % --- 最终输出 ---
    y = y7;

end

%% ===================== 局部函数：预计算滤波器系数 =====================
function [b0, b1, b2, a1, a2] = calc_coeff(wn, wc, k, k2)
    % 连续域：G(s) = (s^2 + wn^2) / (s^2 + 2*wc*s + wn^2)
    % Tustin离散化：s = k*(z-1)/(z+1)
    
    % 连续域系数
    num_b0 = 1; num_b1 = 0; num_b2 = wn^2;
    den_a0 = 1; den_a1 = 2*wc; den_a2 = wn^2;
    
    % 离散化计算
    B0 = num_b0*k2 + num_b1*k + num_b2;
    B1 = 2*num_b2 - 2*num_b0*k2;
    B2 = num_b0*k2 - num_b1*k + num_b2;
    
    A0 = den_a0*k2 + den_a1*k + den_a2;
    A1 = 2*den_a2 - 2*den_a0*k2;
    A2 = den_a0*k2 - den_a1*k + den_a2;
    
    % 归一化（a0=1）
    b0 = B0 / A0;
    b1 = B1 / A0;
    b2 = B2 / A0;
    a1 = A1 / A0;
    a2 = A2 / A0;
end

== matlab function Single_Phase_VSR_Simulation/模仿开关控制1 ==
  data: t input; mod_out output; mod_in input
function mod_out = gate_mod_signal(t, mod_in)
% 功能：0.25s前输出0，0.25s后输出原调制波mod_in
% 输入 t: 仿真时间 (Clock模块)
% 输入 mod_in: 原始调制波信号
% 输出 mod_out: 带使能的调制波信号

t_start = 0.15; % 合闸时间

if t < t_start
    mod_out = 0;          % 合闸前强制输出0
else
    mod_out = mod_in;      % 合闸后输出原调制波
end
end

== matlab function Single_Phase_VSR_Simulation/级联谐波抑制2 ==
  data: u input; y output
function y = Cascade_Notch_Filter(u)
% 级联陷波滤波器：滤除3/5/7次固定频率谐波（150/250/350Hz）
% 输入u：待滤波的标量信号
% 输出y：滤波后的标量信号
% 适配：20kHz采样率（Ts=5e-5），和你的控制环完全对齐

    persistent x3_1 x3_2 x5_1 x5_2 x7_1 x7_2 first_run
    persistent b3_0 b3_1 b3_2 a3_1 a3_2
    persistent b5_0 b5_1 b5_2 a5_1 a5_2
    persistent b7_0 b7_1 b7_2 a7_1 a7_2

    %% ===================== 1. 初始化：仅首次运行 =====================
    if isempty(first_run)
        % --- 固定参数 ---
        Fs = 1e5;          % 采样频率 100kHz
        Ts = 1/Fs;            % 采样周期 5e-5s
        wc = 10;              % 截止角频率 25 rad/s
        
        % 目标谐波频率
        w3 = 2*pi*150;  % 3次谐波 150Hz
        w5 = 2*pi*250;  % 5次谐波 250Hz
        w7 = 2*pi*350;  % 7次谐波 350Hz

        % --- Tustin变换预计算系数 ---
        k = 2/Ts;
        k2 = k*k;

        % --- 3次滤波器系数 ---
        [b3_0, b3_1, b3_2, a3_1, a3_2] = calc_coeff(w3, wc, k, k2);
        % --- 5次滤波器系数 ---
        [b5_0, b5_1, b5_2, a5_1, a5_2] = calc_coeff(w5, wc, k, k2);
        % --- 7次滤波器系数 ---
        [b7_0, b7_1, b7_2, a7_1, a7_2] = calc_coeff(w7, wc, k, k2);

        % --- 显式初始化状态变量为标量 ---
        x3_1 = 0; x3_2 = 0;
        x5_1 = 0; x5_2 = 0;
        x7_1 = 0; x7_2 = 0;
        
        first_run = 1;
    end

    %% ===================== 2. 级联滤波计算（显式差分方程） =====================
    % --- 第1级：3次谐波滤波 ---
    y3 = b3_0*u + x3_1;
    x3_1_next = b3_1*u - a3_1*y3 + x3_2;
    x3_2_next = b3_2*u - a3_2*y3;
    
    % --- 第2级：5次谐波滤波 ---
    y5 = b5_0*y3 + x5_1;
    x5_1_next = b5_1*y3 - a5_1*y5 + x5_2;
    x5_2_next = b5_2*y3 - a5_2*y5;
    
    % --- 第3级：7次谐波滤波 ---
    y7 = b7_0*y5 + x7_1;
    x7_1_next = b7_1*y5 - a7_1*y7 + x7_2;
    x7_2_next = b7_2*y5 - a7_2*y7;
    
    % --- 更新状态变量 ---
    x3_1 = x3_1_next; x3_2 = x3_2_next;
    x5_1 = x5_1_next; x5_2 = x5_2_next;
    x7_1 = x7_1_next; x7_2 = x7_2_next;
    
    % --- 最终输出 ---
    y = y7;

end

%% ===================== 局部函数：预计算滤波器系数 =====================
function [b0, b1, b2, a1, a2] = calc_coeff(wn, wc, k, k2)
    % 连续域：G(s) = (s^2 + wn^2) / (s^2 + 2*wc*s + wn^2)
    % Tustin离散化：s = k*(z-1)/(z+1)
    
    % 连续域系数
    num_b0 = 1; num_b1 = 0; num_b2 = wn^2;
    den_a0 = 1; den_a1 = 2*wc; den_a2 = wn^2;
    
    % 离散化计算
    B0 = num_b0*k2 + num_b1*k + num_b2;
    B1 = 2*num_b2 - 2*num_b0*k2;
    B2 = num_b0*k2 - num_b1*k + num_b2;
    
    A0 = den_a0*k2 + den_a1*k + den_a2;
    A1 = 2*den_a2 - 2*den_a0*k2;
    A2 = den_a0*k2 - den_a1*k + den_a2;
    
    % 归一化（a0=1）
    b0 = B0 / A0;
    b1 = B1 / A0;
    b2 = B2 / A0;
    a1 = A1 / A0;
    a2 = A2 / A0;
end

== matlab function Single_Phase_VSR_Simulation/MATLAB Function1 ==
  data: i_error input; m output
function m  = QPR_Current_Loop(i_error)
% 单相LCL整流器 电流环 多谐振QPR控制器
% 【严格匹配论文公式】G = Kp + Σ(2Kr·wi·s)/(s²+2wi·s + wn²)
% 谐振项：基波50Hz + 3次150Hz +5次250Hz +7次350Hz
% 【参数规则】仅Kp全局共用，Kr/wi/w0 每项独立设置
% 采样率：20kHz | 双线性变换离散化

%% ===================== 独立历史变量 =====================
persistent e1_1 e1_2 m1_1 m1_2  % 基波 n=1
persistent e3_1 e3_2 m3_1 m3_2  % 3次  n=3
persistent e5_1 e5_2 m5_1 m5_2  % 5次  n=5
persistent e7_1 e7_2 m7_1 m7_2  % 7次  n=7

%% ===================== 全局共用参数（仅Kp） =====================
Ts    = 1/20000;   % 采样周期
Kp    = 0.6;       % 【唯一共用参数】比例增益

%% ===================== 各谐振项 独立参数（互不共用） =====================
% === 基波 50Hz (n=1) ===
Kr1 = 55;
wi1 = 15;
w01 = 100*pi;

% === 3次谐波 150Hz (n=3) ===
Kr3 = 150;
wi3 = 6;
w03 = 300*pi;

% === 5次谐波 250Hz (n=5) ===
Kr5 = 55;
wi5 = 6;
w05 = 500*pi;

% === 7次谐波 350Hz (n=7) ===
Kr7 = 55;
wi7 = 6;
w07 = 700*pi;

%% ===================== 初始化 =====================
if isempty(e1_1)
    e1_1=0;e1_2=0;m1_1=0;m1_2=0;
    e3_1=0;e3_2=0;m3_1=0;m3_2=0;
    e5_1=0;e5_2=0;m5_1=0;m5_2=0;
    e7_1=0;e7_2=0;m7_1=0;m7_2=0;
end

%% ===================== 1. 共用比例项 =====================
m_p = Kp * i_error;

%% ===================== 2. 基波谐振项计算 =====================
A1  = 2 * Kr1 * wi1;
B1  = 2 * wi1;
C1  = w01^2;
a0_1 = 4 + 2*B1*Ts + C1*Ts^2;
a1_1 = -8 + 2*C1*Ts^2;
a2_1 = 4 - 2*B1*Ts + C1*Ts^2;
b0_1 =  A1 * Ts;
b1_1 =  0;
b2_1 = -A1 * Ts;
m1 = (b0_1*i_error + b1_1*e1_1 + b2_1*e1_2 - a1_1*m1_1 - a2_1*m1_2) / a0_1;
% 更新
e1_2 = e1_1; e1_1 = i_error;
m1_2 = m1_1; m1_1 = m1;

%% ===================== 3. 3次谐波谐振项计算 =====================
A3  = 2 * Kr3 * wi3;
B3  = 2 * wi3;
C3  = w03^2;
a0_3 = 4 + 2*B3*Ts + C3*Ts^2;
a1_3 = -8 + 2*C3*Ts^2;
a2_3 = 4 - 2*B3*Ts + C3*Ts^2;
b0_3 =  A3 * Ts;
b1_3 =  0;
b2_3 = -A3 * Ts;
m3 = (b0_3*i_error + b1_3*e3_1 + b2_3*e3_2 - a1_3*m3_1 - a2_3*m3_2) / a0_3;
% 更新
e3_2 = e3_1; e3_1 = i_error;
m3_2 = m3_1; m3_1 = m3;

%% ===================== 4. 5次谐波谐振项计算 =====================
A5  = 2 * Kr5 * wi5;
B5  = 2 * wi5;
C5  = w05^2;
a0_5 = 4 + 2*B5*Ts + C5*Ts^2;
a1_5 = -8 + 2*C5*Ts^2;
a2_5 = 4 - 2*B5*Ts + C5*Ts^2;
b0_5 =  A5 * Ts;
b1_5 =  0;
b2_5 = -A5 * Ts;
m5 = (b0_5*i_error + b1_5*e5_1 + b2_5*e5_2 - a1_5*m5_1 - a2_5*m5_2) / a0_5;
% 更新
e5_2 = e5_1; e5_1 = i_error;
m5_2 = m5_1; m5_1 = m5;

%% ===================== 5. 7次谐波谐振项计算 =====================
A7  = 2 * Kr7 * wi7;
B7  = 2 * wi7;
C7  = w07^2;
a0_7 = 4 + 2*B7*Ts + C7*Ts^2;
a1_7 = -8 + 2*C7*Ts^2;
a2_7 = 4 - 2*B7*Ts + C7*Ts^2;
b0_7 =  A7 * Ts;
b1_7 =  0;
b2_7 = -A7 * Ts;
m7 = (b0_7*i_error + b1_7*e7_1 + b2_7*e7_2 - a1_7*m7_1 - a2_7*m7_2) / a0_7;
% 更新
e7_2 = e7_1; e7_1 = i_error;
m7_2 = m7_1; m7_1 = m7;

%% ===================== 总输出叠加 =====================
m = m_p + m1 + m3 + m5 + m7;

%% 可选限幅
% m = min(max(m, -1), 1);
end

== matlab function Single_Phase_VSR_Simulation/MATLAB Function19 ==
  settings: updateMethod=DISCRETE
  data: uin input; alpha output; beta output
function [alpha, beta] = SOGI_FLL_20kHz(uin)
% 严格对应你的 m 文件：20kHz 双线性 PI-FLL
% 输入：uin   单相电压
% 输出：alpha 同相输出 uα = x2
%      beta  正交输出 uβ = omega0*x3

%% 固定参数（和你的m文件完全一致）
dt = 5e-5;
K  = 1.414;
K1 = 0.25;
gamma_p =30;
gamma_i =500;
w_max = 2*pi*60;
w_min = 2*pi*40;

%% 状态持久化
persistent x1_prev x2_prev x3_prev omega0_prev U_prev integral_f first_run;
if isempty(first_run)
    x1_prev = 0;
    x2_prev = 0;
    x3_prev = 0;
    omega0_prev = 2*pi*50;
    U_prev = uin;
    integral_f = 0;
    first_run = false;
end

%% 1. 当前输入
U_curr = uin;
omega0_prev_local = omega0_prev;

%% 2. 频率预畸变
omega_pre = (2/dt) * tan(omega0_prev_local * dt / 2);

%% 3. 状态矩阵 A, B
A_mat = [
    -K1*omega_pre, -K1*omega_pre, 0;
    -K*omega_pre,  -K*omega_pre,  -omega_pre^2;
    0,              1,              0
];
B_mat = [
    K1*omega_pre;
    K*omega_pre;
    0
];

%% 4. 双线性变换
I_mat = eye(3);
M1 = I_mat - (dt/2)*A_mat;
M2 = I_mat + (dt/2)*A_mat;
U_avg = U_curr + U_prev;

x_prev_vec = [x1_prev; x2_prev; x3_prev];
x_curr_vec = M1 \ (M2 * x_prev_vec + (dt/2)*B_mat * U_avg);

x1_curr = x_curr_vec(1);
x2_curr = x_curr_vec(2);
x3_curr = x_curr_vec(3);

%% 5. PI-FLL 频率环
deltaU = U_curr - x1_curr - x2_curr;
deltaU_prime_val = omega0_prev_local * x3_curr;
epsilon_f = deltaU * deltaU_prime_val;

integral_f = integral_f + epsilon_f * dt;
domega0dt = -gamma_p * epsilon_f - gamma_i * integral_f;
omega0_curr = omega0_prev_local + dt * domega0dt;

% 频率限幅
omega0_curr = max(min(omega0_curr, w_max), w_min);

%% 6. 输出 alpha beta
alpha = x2_curr;
beta  = omega0_curr * x3_curr;

%% 7. 更新状态
x1_prev = x1_curr;
x2_prev = x2_curr;
x3_prev = x3_curr;
omega0_prev = omega0_curr;
U_prev = U_curr;

end

== matlab function Single_Phase_VSR_Simulation/MATLAB Function3 ==
  data: u_alpha input; theta output; u_beta input; qerror output
function [theta, qerror] = SRF_PLL(u_alpha, u_beta)
% 同步旋转坐标系锁相环 SRF-PLL
% 【已修改为：纯自适应频率版本 → 和你主循环PLL完全一致】
% 输入：u_alpha, u_beta
% 输出：theta 锁相相位, qerror q分量（趋近0）

    %% ===================== 1. 固定参数 =====================
    Ts = 5e-5;               % 20kHz 采样步长（必须匹配）
    
    % PI参数（和你主循环一致）
    kp_pll = 200;
    ki_pll = 7000;

    %% ===================== 2. 持久变量 =====================
    persistent theta_prev
    persistent integral_pll
    
    if isempty(theta_prev)
        theta_prev = 0;
        integral_pll = 0;
    end

    %% ===================== 3. Park 变换 =====================
    cos_theta = cos(theta_prev);
    sin_theta = sin(theta_prev);
    
    u_d =  u_alpha * cos_theta + u_beta * sin_theta;
    u_q = -u_alpha * sin_theta + u_beta * cos_theta;
    
    qerror = u_q;  % q分量（锁相成功→0）

    %% ===================== 4. PI控制器（我的版本：直接输出ω） =====================
    integral_pll = integral_pll + qerror * Ts;          % 积分
    omega_pll    = kp_pll * qerror + ki_pll * integral_pll; % 直接输出角频率

    %% ===================== 5. 积分生成相位 =====================
    theta = theta_prev + omega_pll * Ts;

    %% ===================== 6. 相位归一化（±π） =====================
    if theta > pi
        theta = theta - 2*pi;
    elseif theta < -pi
        theta = theta + 2*pi;
    end

    %% ===================== 7. 更新状态 =====================
    theta_prev = theta;
end

== matlab function Single_Phase_VSR_Simulation/MATLAB Function15 ==
  data: IGm_total input; Igm_clean output
function Igm_clean = Notch_100Hz_IGm(IGm_total)
% 100Hz陷波滤波器，放在IGm求和后，滤除二次纹波
% 陷波频率100Hz，带宽6Hz，采样率20kHz
% 输入：IGm_total = IGm1 + IGm2
% 输出：Igm_clean = 滤除100Hz纹波后的纯直流信号

%% 历史变量
persistent x_prev1 x_prev2 y_prev1 y_prev2;

%% 固定参数
Ts = 1/20000;
f0 = 100;          % 陷波频率100Hz
bw = 6;            % 陷波带宽6Hz
w0 = 2*pi*f0;
wb = 2*pi*bw;

%% 双线性变换离散化系数
k = 2/Ts;
a0 = k^2 + wb*k + w0^2;
a1 = 2*(w0^2 - k^2);
a2 = k^2 - wb*k + w0^2;
b0 = k^2 + w0^2;
b1 = 2*(w0^2 - k^2);
b2 = k^2 + w0^2;

%% 归一化
b0 = b0/a0;
b1 = b1/a0;
b2 = b2/a0;
a1 = a1/a0;
a2 = a2/a0;

%% 初始化
if isempty(x_prev1)
    x_prev1 = 0; x_prev2 = 0;
    y_prev1 = 0; y_prev2 = 0;
end

%% 差分方程
Igm_clean = b0*IGm_total + b1*x_prev1 + b2*x_prev2 - a1*y_prev1 - a2*y_prev2;

%% 更新历史变量
x_prev2 = x_prev1;
x_prev1 = IGm_total;
y_prev2 = y_prev1;
y_prev1 = Igm_clean;

end

== matlab function Single_Phase_VSR_Simulation/模仿开关控制 ==
  data: t input; mod_out output; mod_in input
function mod_out = gate_mod_signal(t, mod_in)
% 功能：0.25s前输出0，0.25s后输出原调制波mod_in
% 输入 t: 仿真时间 (Clock模块)
% 输入 mod_in: 原始调制波信号
% 输出 mod_out: 带使能的调制波信号

t_start = 0.15; % 合闸时间

if t < t_start
    mod_out = 0;          % 合闸前强制输出0
else
    mod_out = mod_in;      % 合闸后输出原调制波
end
end

== matlab function Single_Phase_VSR_Simulation/MATLAB Function16 ==
  data: alpha input; d output; beta input; theta input; q output
function [d, q] = Park_Transform(alpha, beta, theta)
% Park变换模块（直接输入SOGI-FLL的theta，无内部积分）
% 输入：
%   alpha - α轴分量（SOGI-FLL的U_prime）
%   beta  - β轴分量（SOGI-FLL的deltaU_prime）
%   theta - 瞬时相位（SOGI-FLL直接输出的theta）
% 输出：
%   d         - d轴（直轴）分量
%   q         - q轴（交轴）分量
%   cos_theta - 相位θ的余弦值（新增输出）
%   sin_theta - 相位θ的正弦值（新增输出）

%% 核心计算
cos_theta = cos(theta);  % 相位θ的余弦值
sin_theta = sin(theta);  % 相位θ的正弦值


% 修正后的 Park 变换公式（d轴对齐同相分量 beta）
d =  alpha * cos_theta + beta * sin_theta;
q = -alpha * sin_theta + beta * cos_theta;
end
